simulink model "question9_2018b"  (R2020b)
settings: Solver=VariableStepAuto  StartTime=0.0  StopTime=100  RelTol=1e-3
values from neighbouring files (symbols this model uses):
  D = 0    [Alt_Industrial_plant.m]    (also in IndustrialPlant.m = [0;     0;     0;     0]; OldProject.m = [0;0]; observerWorkingExample.m)
  Jd = 0.0025    [Alt_Industrial_plant.m]    (also in IndustrialPlant.m)
  K = acker(A,B,des_poles)    [Alt_Industrial_plant.m]    (also in IndustrialPlant.m = place(A,B, [p1, p2, p3, p4]); ObserverExample.m = place(A,B,[p1 p2 p3]); OldProject.m = place(A,B,Pole_fb); observerWorkingExample.m)
libraries: pid_lib x1
settings Model: Creator=Dimitri  LastModifiedBy=Yaipiti
settings DataIOCC: ReturnWorkspaceOutputs=off
settings DebuggingCC: ArithmeticOperatorsInVariantConditions=warning
settings SFSimCC: CustomCodeUndefinedFunction=UseInterfaceOnly

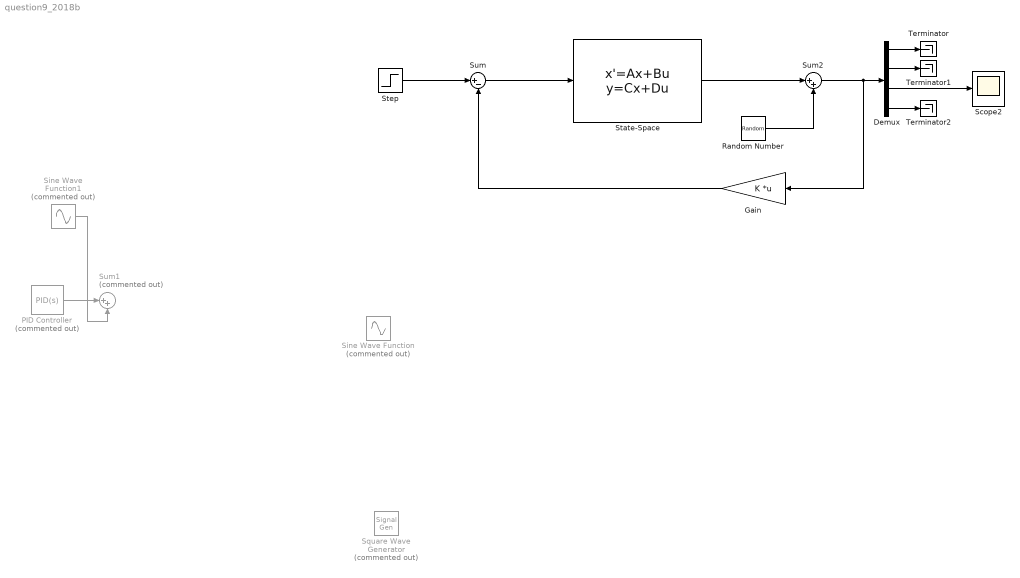
== system question9_2018b ==
  Demux : Demux
  Gain : Gain  Gain=K  Multiplication=Matrix(K*u) (u vector)
  PID Controller : pid_lib/PID Controller  Commented=on  Controller=PID  Form=Parallel  TimeDomain=Continuous-time  UseExternalTs=off  SampleTime=-1  IntegratorMethod=Forward Euler  FilterMethod=Forward Euler  ControllerParametersSource=internal  P=0.0109489475340948  I=0.0306597041287344  D=-0.00168563737676081  UseFilter=on  N=5.71917457059038  TunerSelectOption=Transfer Function Based (PID Tuner App)  InitialConditionSource=internal  InitialConditionForIntegrator=0  InitialConditionForFilter=0  DifferentiatorICPrevScaledInput=0  ExternalReset=none  TrackingMode=off  Kt=1  LimitOutput=off  SatLimitsSource=internal  UpperSaturationLimit=inf  LowerSaturationLimit=-inf  LinearizeAsGain=on  AntiWindupMode=none  Kb=1  POutMin=[]  POutMax=[]  IOutMin=[]  IOutMax=[]  DOutMin=[]  DOutMax=[]  NOutMin=[]  NOutMax=[]  SumOutMin=[]  SumOutMax=[]  SaturationOutMin=[]  SaturationOutMax=[]  PParamMin=[]  PParamMax=[]  IParamMin=[]  IParamMax=[]  DParamMin=[]  DParamMax=[]  NParamMin=[]  NParamMax=[]  KbParamMin=[]  KbParamMax=[]  KtParamMin=[]  KtParamMax=[]  KbOutMin=[]  KbOutMax=[]  KtOutMin=[]  KtOutMax=[]  IntegratorOutMin=[]  IntegratorOutMax=[]  FilterOutMin=[]  FilterOutMax=[]  SumI1OutMin=[]  SumI1OutMax=[]  SumI2OutMin=[]  SumI2OutMax=[]  SumI3OutMin=[]  SumI3OutMax=[]  SumI4OutMin=[]  SumI4OutMax=[]  SumDOutMin=[]  SumDOutMax=[]  DifferentiatorOutMin=[]  DifferentiatorOutMax=[]  FilterDiffOutCoefMin=[]  FilterDiffOutCoefMax=[]  ReciprocalOutMin=[]  ReciprocalOutMax=[]  SumDenOutMin=[]  SumDenOutMax=[]  SumNumOutMin=[]  SumNumOutMax=[]  DivideOutMin=[]  DivideOutMax=[]  UdiffTsProdOutMin=[]  UdiffTsProdOutMax=[]  NTsProdOutMin=[]  NTsProdOutMax=[]  UintegralTsProdOutMin=[]  UintegralTsProdOutMax=[]  UngainTsProdOutMin=[]  UngainTsProdOutMax=[]  IntegratorContinuousStateAttributes=''  IntegratorStateMustResolveToSignalObject=off  IntegratorRTWStateStorageClass=Auto  FilterContinuousStateAttributes=''  FilterStateMustResolveToSignalObject=off  FilterRTWStateStorageClass=Auto  ParallelPVariant=InternalParameters  IdealPVariant=Disabled  IVariant=InternalParameters  DVariant=InternalParameters  IntegratorVariant=Continuous  SatVariant=Disabled  AWVariant=Passthrough  PCopyVariant=Disabled  TRVariant=Disabled  FdbkBlocksVariant=Forward  IdealPFdbkVariant=Disabled  SatFdbkVariant=Disabled  DerivativeFilterVariant=ContFilter  NVariant=InternalParameters  NCopyVariant=Disabled  FilterICVariant=InternalICsFilter  IntegratorICVariant=InternalICs  ExternalResetVariant=Disabled  TRSumVariant=Passthrough  SumFdbkVariant=Disabled  SumVariant=Sum_PID  TsampFilterVariant=InternalTs  TsampNgainVariant=Passthrough  TsampIntegralVariant=Passthrough  ExternalSaturationOutDataTypeStr=Inherit: Same as second input
  Random Number : RandomNumber  Variance=0.00001  SampleTime=0.1
  Scope2 : Scope
  Sine Wave Function : Sin  Commented=on  Amplitude=2  Frequency=0.1  SampleTime=0
  Sine Wave Function1 : Sin  Commented=on  Amplitude=0.001  Frequency=0.00001  SampleTime=0
  Square Wave Generator : SignalGenerator  Commented=on  WaveForm=square  Amplitude=5  Units=rad/sec
  State-Space : StateSpace  A=|  B=[0; 1/Jd; 0; 0]  C=eye(4)  D=D  InitialCondition=0
      | [ 0 1 0 0;
      |     (-k*(gr)^(-2))/Jd  -c1/Jd  (k*(gr)^(-1))/Jd  0;
      |       0 0 0 1;
      |      (k*(gr)^(-1))/J1  0 -k/J1 -c2/J1]
  Step : Step  SampleTime=0
  Sum : Sum  Inputs=|+-
  Sum1 : Sum  Commented=on  Inputs=|++
  Sum2 : Sum  Inputs=|++
  Terminator : Terminator
  Terminator1 : Terminator
  Terminator2 : Terminator
  wires:
  PID Controller/1 -> Sum1/1
  Sine Wave Function1/1 -> Sum1/2
  Sum/1 -> State-Space/1
  Gain/1 -> Sum/2
  Random Number/1 -> Sum2/2
  State-Space/1 -> Sum2/1
  Sum2/1 -> Gain/1, Demux/1
  Demux/1 -> Terminator/1
  Demux/4 -> Terminator2/1
  Demux/2 -> Terminator1/1
  Demux/3 -> Scope2/1
  Step/1 -> Sum/1
